simulink model "FWDKinematics"  (R2020a)
settings: Solver=FixedStepAuto  StartTime=0.0  StopTime=t_final  FixedStep=dt  RelTol=1e-3
settings Model: Creator=m2aali  LastModifiedBy=m2aali

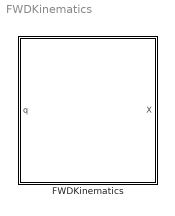
== system FWDKinematics ==
  FWDKinematics : Subsystem

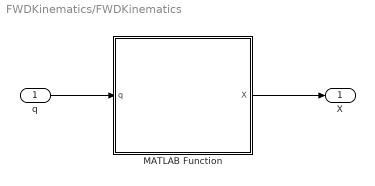
== system FWDKinematics/FWDKinematics ==
  q : Inport
  MATLAB Function : MATLAB Function  TreatAsAtomicUnit=on
  X : Outport
  wires:
  MATLAB Function/1(X) -> X/1
  q/1 -> MATLAB Function/1(q)

== matlab function FWDKinematics/MATLAB Function ==
  data: q input; X output
function X = FWDKinematics(q)
%%% Forward Kinematic Function


%% Joint Space variables
% q is 3*1 vector of joint variables (radian), q = [q1;q2;q3]
q1 = q(1);
q2 = q(2);
q3 = q(3);

%% general physical parameters
l1 = 0.6731;
l2 = 0.432;
l3 = 0.434;
lc2 = 0.216;
lc3 = 0.164;

%% Forward Kinematic
% X is 3*1 vecto of end-effector position in task space, X = [x;y;z]

x = cos(q1) * (l2 * cos(q2) + l3 * sin(q2 + q3));
y = sin(q1) * (l2 * cos(q2) + l3 * sin(q2 + q3));
z = l1 - l2 * sin(q2) + l3 * cos(q2 + q3);

X = [x;y;z]
